simulink model "modelo_NL"  (R2018a)
settings: Solver=VariableStepAuto  StartTime=0.0  StopTime=0.5  MaxStep=1e-4  RelTol=1e-3
values from neighbouring files (symbols this model uses):
  alpha_Cu = 3.9e-3    (= 0.0039)    [proyecto_global_integrador.m]
  b_eq = b_m + b_l/r^2    (= 1.5e-05)    [proyecto_global_integrador.m]
  C_ts = 1.091    [proyecto_global_integrador.m]
  J_eq = J_m + J_l/r^2    (= 5.65099476805e-06)    [proyecto_global_integrador.m]
  L_d = 6.6e-3    (= 0.0066)    [proyecto_global_integrador.m]
  L_ls = 0.8e-3    (= 0.0008)    [proyecto_global_integrador.m]
  L_q = 5.8e-3    (= 0.0058)    [proyecto_global_integrador.m]
  lambda_m = 0.01546    [proyecto_global_integrador.m]
  P_p = 3    [proyecto_global_integrador.m]
  r = 314.3008    [proyecto_global_integrador.m]
  R_s = 1.02    [polos_choreo_no_se_puede_robar_mas_con_esto.m]    (also in proyecto_global_integrador.m)
  R_tsamb = 55    [proyecto_global_integrador.m]
  T_ambmax = 40    [proyecto_global_integrador.m]
libraries: peTransforms x2
settings Model: Creator=gabrielq  LastModifiedBy=gabrielq

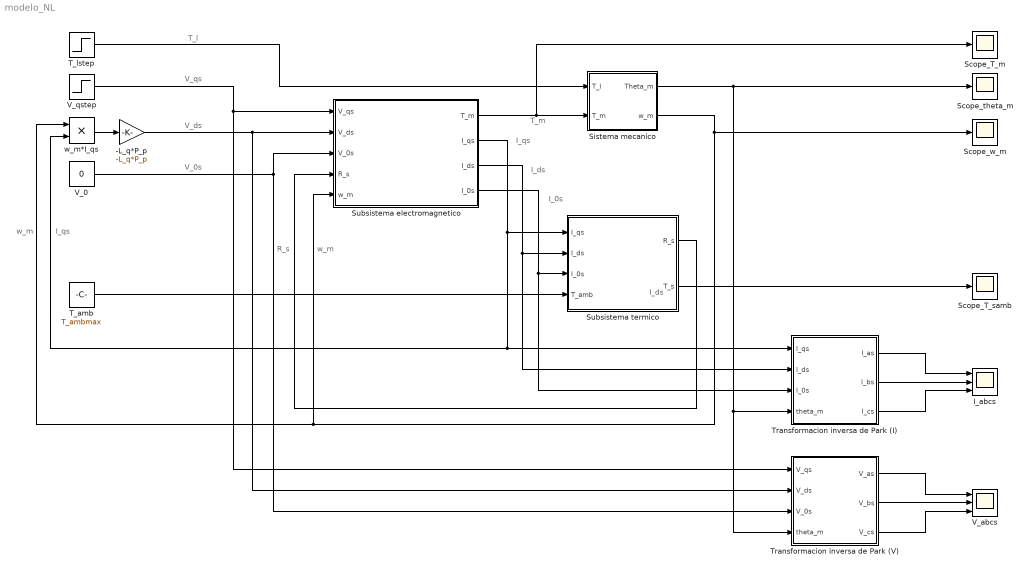
== system modelo_NL ==
  note: I_ds
  note: V_0s
  note: V_ds
  note: T_l
  note: V_qs
  note: T_m
  note: R_s
  note: I_0s
  note: I_ds
  note: I_qs
  note: w_m
  note: I_qs
  note: w_m
  -L_q*P_p : Gain  Gain=-L_q*P_p
  I_abcs : Scope  NumInputPorts=3
  Scope_T_m : Scope
  Scope_T_samb : Scope
  Scope_theta_m : Scope
  Scope_w_m : Scope
  Sistema mecanico : Subsystem
  Subsistema electromagnetico : Subsystem
  Subsistema termico : Subsystem
  T_amb : Constant  Value=T_ambmax
  T_lstep : Step  Time=0.3  After=1.57  SampleTime=0
  Transformacion inversa de Park (I) : Subsystem
  Transformacion inversa de Park (V) : Subsystem
  V_0 : Constant  Value=0
  V_abcs : Scope  NumInputPorts=3
  V_qstep : Step  Time=0.1  After=19.596  SampleTime=0
  w_m*I_qs : Product
  wires:
  w_m*I_qs/1 -> -L_q*P_p/1
  -L_q*P_p/1 -> Transformacion inversa de Park (V)/2(V_ds), Subsistema electromagnetico/2(V_ds)
  V_qstep/1 -> Transformacion inversa de Park (V)/1(V_qs), Subsistema electromagnetico/1(V_qs)
  V_0/1 -> Transformacion inversa de Park (V)/3(V_0s), Subsistema electromagnetico/3(V_0s)
  Subsistema electromagnetico/2(I_qs) -> Subsistema termico/1(I_qs), w_m*I_qs/2, Transformacion inversa de Park (I)/1(I_qs)
  Subsistema electromagnetico/3(I_ds) -> Transformacion inversa de Park (I)/2(I_ds), Subsistema termico/2(I_ds)
  Subsistema electromagnetico/4(I_0s) -> Transformacion inversa de Park (I)/3(I_0s), Subsistema termico/3(I_0s)
  Subsistema electromagnetico/1(T_m) -> Sistema mecanico/2(T_m), Scope_T_m/1
  Sistema mecanico/2(w_m) -> Subsistema electromagnetico/5(w_m), w_m*I_qs/1, Scope_w_m/1
  Sistema mecanico/1(Theta_m) -> Scope_theta_m/1, Transformacion inversa de Park (V)/4(theta_m), Transformacion inversa de Park (I)/4(theta_m)
  T_lstep/1 -> Sistema mecanico/1(T_l)
  Subsistema termico/2(T_s) -> Scope_T_samb/1
  T_amb/1 -> Subsistema termico/4(T_amb)
  Subsistema termico/1(R_s) -> Subsistema electromagnetico/4(R_s)
  Transformacion inversa de Park (I)/1(I_as) -> I_abcs/1
  Transformacion inversa de Park (I)/2(I_bs) -> I_abcs/2
  Transformacion inversa de Park (I)/3(I_cs) -> I_abcs/3
  Transformacion inversa de Park (V)/1(V_as) -> V_abcs/1
  Transformacion inversa de Park (V)/2(V_bs) -> V_abcs/2
  Transformacion inversa de Park (V)/3(V_cs) -> V_abcs/3

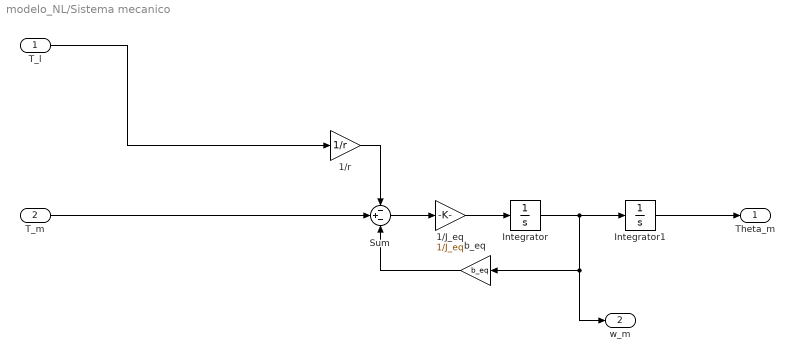
== system modelo_NL/Sistema mecanico ==
  T_l : Inport
  T_m : Inport  Port=2
  1/J_eq : Gain  Gain=1/J_eq
  1/r : Gain  Gain=1/r
  Integrator : Integrator
  Integrator1 : Integrator
  Sum : Sum  Inputs=-+-
  b_eq : Gain  Gain=b_eq
  Theta_m : Outport
  w_m : Outport  Port=2
  wires:
  b_eq/1 -> Sum/3
  1/J_eq/1 -> Integrator/1
  T_l/1 -> 1/r/1
  Integrator1/1 -> Theta_m/1
  Sum/1 -> 1/J_eq/1
  T_m/1 -> Sum/2
  Integrator/1 -> Integrator1/1, w_m/1, b_eq/1
  1/r/1 -> Sum/1

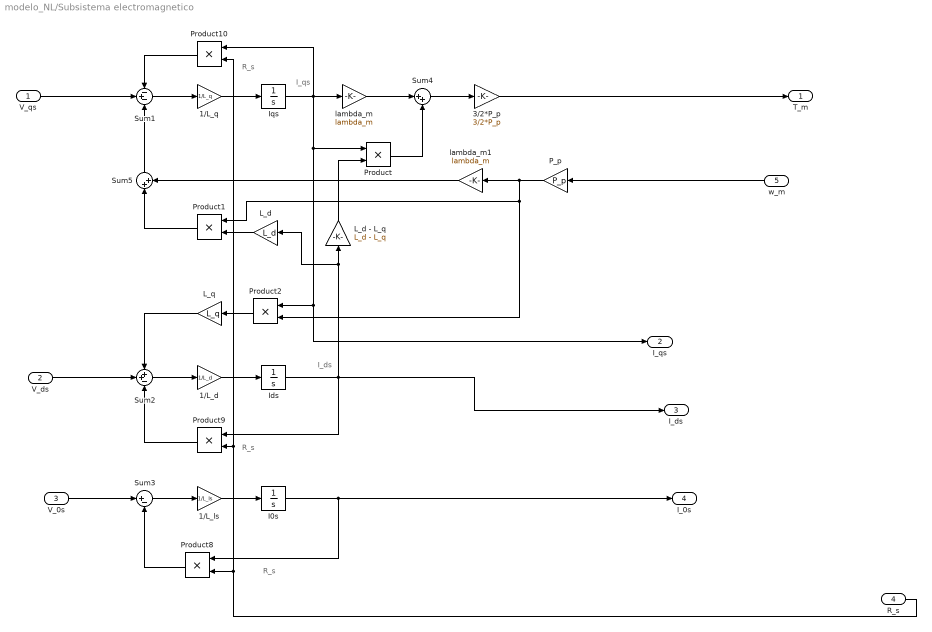
== system modelo_NL/Subsistema electromagnetico ==
  note: I_ds
  note: I_qs
  note: R_s
  note: R_s
  note: R_s
  V_qs : Inport
  V_ds : Inport  Port=2
  V_0s : Inport  Port=3
  R_s : Inport  Port=4
  w_m : Inport  Port=5
  1/L_d : Gain  Gain=1/L_d
  1/L_ls : Gain  Gain=1/L_ls
  1/L_q : Gain  Gain=1/L_q
  3/2*P_p : Gain  Gain=3/2*P_p
  I0s : Integrator
  Ids : Integrator
  Iqs : Integrator
  L_d : Gain  Gain=L_d
  L_d - L_q : Gain  Gain=L_d - L_q
  L_q : Gain  Gain=L_q
  P_p : Gain  Gain=P_p
  Product{,1..2,8..10} (6 alike) : Product
  Sum1 : Sum  Inputs=-+-
  Sum2 : Sum  Inputs=++-
  Sum3 : Sum  Inputs=|+-
  Sum4 : Sum  Inputs=|++
  Sum5 : Sum  Inputs=|++
  lambda_m : Gain  Gain=lambda_m
  lambda_m1 : Gain  Gain=lambda_m
  T_m : Outport
  I_qs : Outport  Port=2
  I_ds : Outport  Port=3
  I_0s : Outport  Port=4
  wires:
  Sum2/1 -> 1/L_d/1
  V_ds/1 -> Sum2/2
  I0s/1 -> I_0s/1, Product8/1
  1/L_ls/1 -> I0s/1
  L_d/1 -> Product1/2
  w_m/1 -> P_p/1
  R_s/1 -> Product10/2, Product9/2, Product8/2
  P_p/1 -> lambda_m1/1, Product2/2, Product1/1
  L_d - L_q/1 -> Product/2
  Sum5/1 -> Sum1/3
  Product8/1 -> Sum3/2
  Sum3/1 -> 1/L_ls/1
  V_0s/1 -> Sum3/1
  Ids/1 -> I_ds/1, L_d/1, L_d - L_q/1, Product9/1
  Sum1/1 -> 1/L_q/1
  Product10/1 -> Sum1/1
  Iqs/1 -> I_qs/1, Product2/1, Product/1, Product10/1, lambda_m/1
  Product/1 -> Sum4/2
  L_q/1 -> Sum2/1
  V_qs/1 -> Sum1/2
  Product1/1 -> Sum5/1
  lambda_m1/1 -> Sum5/2
  Sum4/1 -> 3/2*P_p/1
  1/L_d/1 -> Ids/1
  3/2*P_p/1 -> T_m/1
  1/L_q/1 -> Iqs/1
  Product9/1 -> Sum2/3
  lambda_m/1 -> Sum4/1
  Product2/1 -> L_q/1

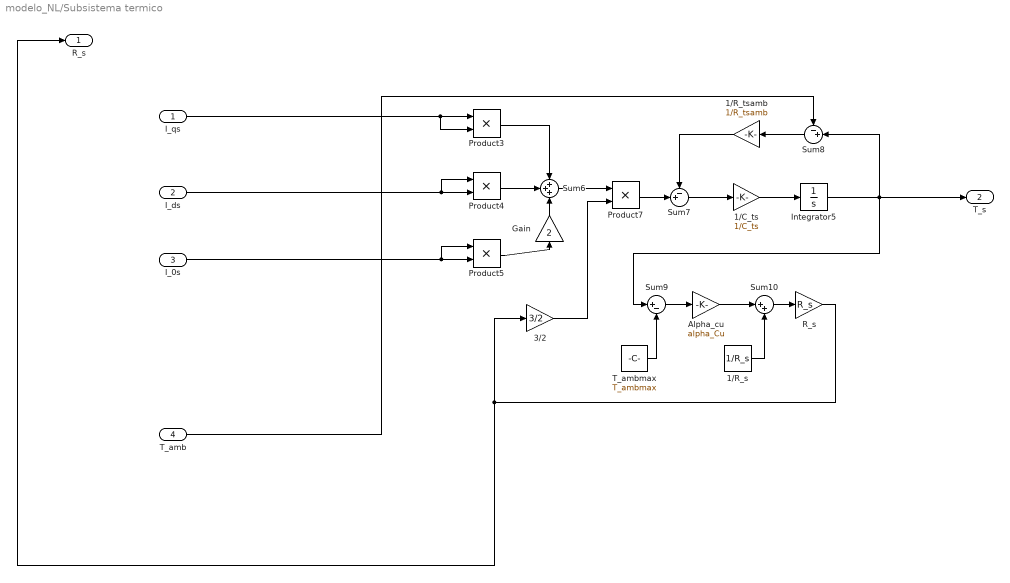
== system modelo_NL/Subsistema termico ==
  I_qs : Inport
  I_ds : Inport  Port=2
  I_0s : Inport  Port=3
  T_amb : Inport  Port=4
  1/C_ts : Gain  Gain=1/C_ts
  "1/R_s " : Constant  Value=1/R_s
  1/R_tsamb : Gain  Gain=1/R_tsamb
  "3/2 " : Gain  Gain=3/2
  "Alpha_cu " : Gain  Gain=alpha_Cu
  Gain : Gain  Gain=2
  Integrator5 : Integrator
  Product{3..5,7} (4 alike) : Product
  "R_s " : Gain  Gain=R_s
  Sum10 : Sum  Inputs=|++
  Sum6 : Sum  Inputs=+++
  Sum7 : Sum  Inputs=-+|
  Sum8 : Sum  Inputs=-+|
  Sum9 : Sum  Inputs=|+-
  "T_ambmax " : Constant  Value=T_ambmax
  R_s : Outport
  T_s : Outport  Port=2
  wires:
  Product4/1 -> Sum6/2
  Product3/1 -> Sum6/1
  1/R_tsamb/1 -> Sum7/1
  Sum6/1 -> Product7/1
  "3/2 "/1 -> Product7/2
  Sum8/1 -> 1/R_tsamb/1
  I_ds/1 -> Product4/2, Product4/1
  Sum7/1 -> 1/C_ts/1
  Product7/1 -> Sum7/2
  "1/R_s "/1 -> Sum10/2
  I_qs/1 -> Product3/2, Product3/1
  I_0s/1 -> Product5/1, Product5/2
  Gain/1 -> Sum6/3
  "T_ambmax "/1 -> Sum9/2
  T_amb/1 -> Sum8/1
  Sum9/1 -> "Alpha_cu "/1
  Sum10/1 -> "R_s "/1
  1/C_ts/1 -> Integrator5/1
  Product5/1 -> Gain/1
  "Alpha_cu "/1 -> Sum10/1
  "R_s "/1 -> R_s/1, "3/2 "/1
  Integrator5/1 -> T_s/1, Sum8/2, Sum9/1

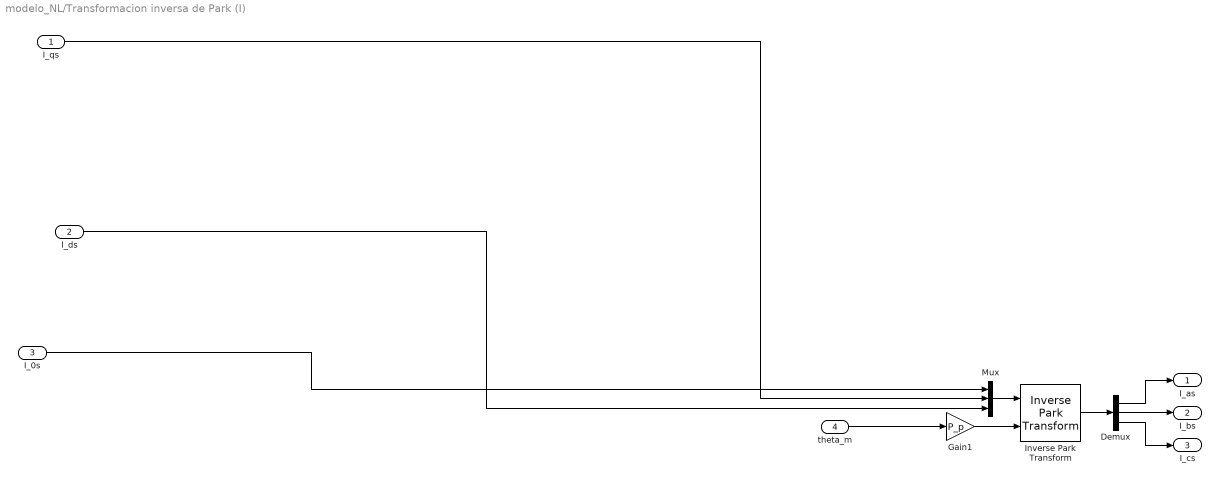
== system modelo_NL/Transformacion inversa de Park (I) ==
  I_qs : Inport
  I_ds : Inport  Port=2
  I_0s : Inport  Port=3
  theta_m : Inport  Port=4
  Demux : Demux  Outputs=3
  Gain1 : Gain  Gain=P_p
  Inverse Park Transform : peTransforms/Inverse Park Transform  AxisAlignment=Q-axis  PowerInvariant=off
  Mux : Mux  Inputs=3
  I_as : Outport
  I_bs : Outport  Port=2
  I_cs : Outport  Port=3
  wires:
  I_qs/1 -> Mux/2
  Mux/1 -> Inverse Park Transform/1
  Gain1/1 -> Inverse Park Transform/2
  Inverse Park Transform/1 -> Demux/1
  theta_m/1 -> Gain1/1
  I_ds/1 -> Mux/3
  Demux/2 -> I_bs/1
  Demux/1 -> I_as/1
  Demux/3 -> I_cs/1
  I_0s/1 -> Mux/1

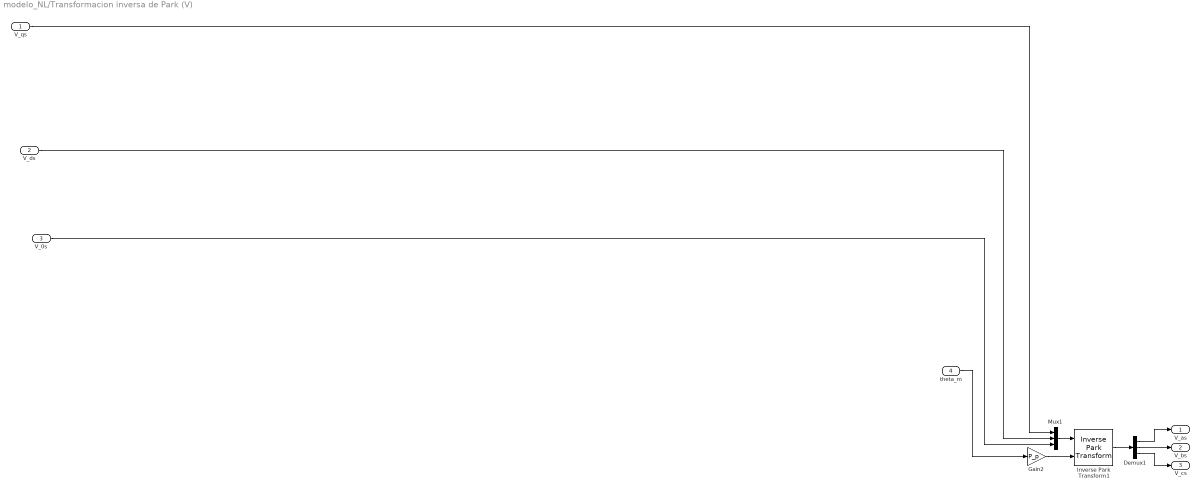
== system modelo_NL/Transformacion inversa de Park (V) ==
  V_qs : Inport
  V_ds : Inport  Port=2
  V_0s : Inport  Port=3
  theta_m : Inport  Port=4
  Demux1 : Demux  Outputs=3
  Gain2 : Gain  Gain=P_p
  Inverse Park Transform1 : peTransforms/Inverse Park Transform  AxisAlignment=Q-axis  PowerInvariant=off
  Mux1 : Mux  Inputs=3
  V_as : Outport
  V_bs : Outport  Port=2
  V_cs : Outport  Port=3
  wires:
  theta_m/1 -> Gain2/1
  Gain2/1 -> Inverse Park Transform1/2
  V_ds/1 -> Mux1/2
  V_qs/1 -> Mux1/1
  Inverse Park Transform1/1 -> Demux1/1
  Demux1/3 -> V_cs/1
  Demux1/2 -> V_bs/1
  Mux1/1 -> Inverse Park Transform1/1
  V_0s/1 -> Mux1/3
  Demux1/1 -> V_as/1
